simulink model "ctrl_student"  (R2020b)
settings: Solver=FixedStepAuto  StartTime=0.0  StopTime=Inf  FixedStep=0.01  RelTol=1e-3  EnableMultiTasking=on
model workspace (MAT data in the model file):
  SL_ROS_VariableLengthArrays_MaxSizes.CommonInfo.ArrayTruncateAction = 'EmitWarning'
  SL_ROS_VariableLengthArrays_MaxSizes.MsgTypeMap = containers.Map
  SL_ROS_VariableLengthArrays_MaxSizes.MsgTypeMap.serialization.keys = {'std_msgs/MultiArrayDimension', 'std_msgs/MultiArrayLayout'}
  SL_ROS_VariableLengthArrays_MaxSizes.MsgTypeMap.serialization.values{1}.PropertyName = 'Label'
  SL_ROS_VariableLengthArrays_MaxSizes.MsgTypeMap.serialization.values{1}.DataType = 'uint8'
  SL_ROS_VariableLengthArrays_MaxSizes.MsgTypeMap.serialization.values{1}.MaxLength = 2
  SL_ROS_VariableLengthArrays_MaxSizes.MsgTypeMap.serialization.values{2}.PropertyName = 'Dim'
  SL_ROS_VariableLengthArrays_MaxSizes.MsgTypeMap.serialization.values{2}.DataType = 'std_msgs/MultiArrayDimension'
  SL_ROS_VariableLengthArrays_MaxSizes.MsgTypeMap.serialization.values{2}.MaxLength = 1
  SL_ROS_VariableLengthArrays_MaxSizes.MsgTypeMap.serialization.uniformity = 0
  SL_ROS_VariableLengthArrays_MaxSizes.MsgTypeMap.serialization.keyType = 'char'
  SL_ROS_VariableLengthArrays_MaxSizes.MsgTypeMap.serialization.valueType = 'any'
undefined symbols (not defined in the file): Data, Data_SL_Info, Layout, X, Y, Z
libraries: robotlib x12
settings Model: SimulationMode=external  ExtModeEnableFloating=off  Creator=erlendbasso  LastModifiedBy=erlendbasso
settings SolverCC: PositivePriorityOrder=on
settings OptimizationCC: EnhancedBackFolding=on  PassReuseOutputArgsAs=Individual arguments  ZeroExternalMemoryAtStartup=off  ZeroInternalMemoryAtStartup=off  MaxStackSize=64  OptimizeBlockOrder=speed  DifferentSizesBufferReuse=on  OptimizationCustomize=off  EfficientTunableParamExpr=on
settings DebuggingCC: ParameterTunabilityLossMsg=error
settings HardwareCC: ProdBitPerPointer=32  ProdBitPerSizeT=32  ProdBitPerPtrDiffT=32  ProdLargestAtomicInteger=Long  ProdLargestAtomicFloat=Double  ProdWordSize=32  ProdHWDeviceType=ARM Compatible->ARM Cortex
settings RTWCC: Description=Embedded Coder  SystemTargetFile=ert.tlc  HardwareBoard=Raspberry Pi - Robot Operating System (ROS)  TLCOptions="-aInlineSetEventsForThisBaseRateFcn=TLC_FALSE -aSuppressMultiTaskScheduler=TLC_FALSE  -aRateBasedStepFcn=0"  TemplateMakefile=ert_default_tmf  Toolchain=Catkin  BuildConfiguration=Faster Runs  TargetLang=C++
settings CodeAppCC: ForceParamTrailComments=on  IgnoreCustomStorageClasses=off  OperatorAnnotations=on  SimulinkDataObjDesc=on  SFDataObjDesc=on  InsertBlockDesc=on
settings ERTTargetCC: SupportContinuousTime=on  SupportVariableSizeSignals=on  ExtModeTransport=2  ExtModeMexFile=ext_xcp  ExtModeIntrfLevel=Level2 - Open

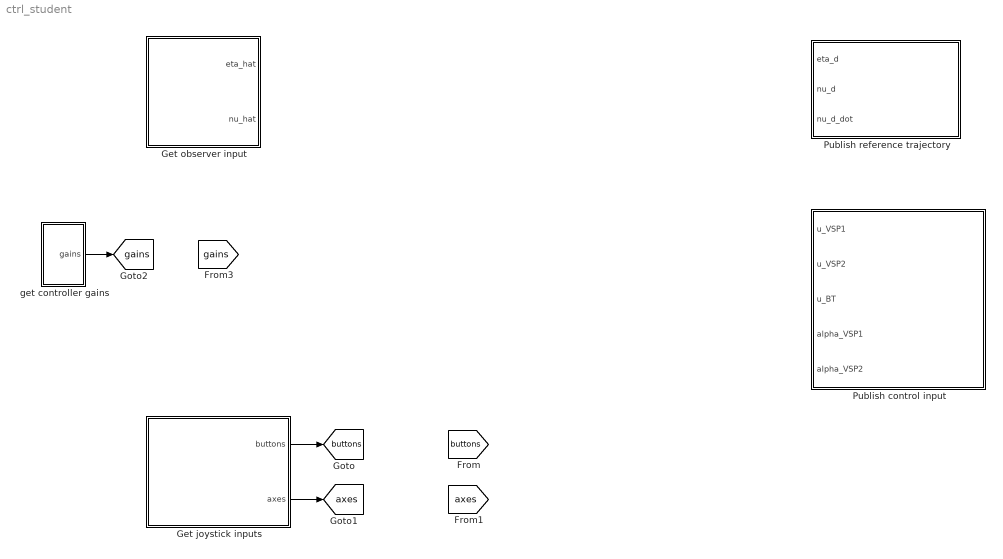
== system ctrl_student ==
  Get joystick inputs : Subsystem
  Get observer input : Subsystem
  Publish control input : Subsystem
  Publish reference trajectory : Subsystem
  get controller gains : Subsystem
  tag scope: axes=global, buttons=global, gains=global
  wires:
  Get joystick inputs/2(axes) -> [axes]
  Get joystick inputs/1(buttons) -> [buttons]
  get controller gains/1(gains) -> [gains]

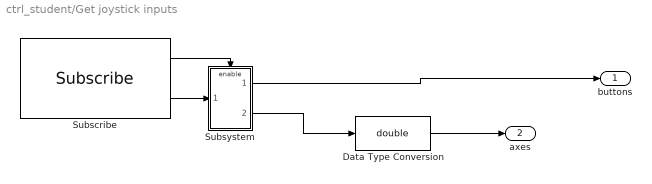
== system ctrl_student/Get joystick inputs ==
  Data Type Conversion : DataTypeConversion  OutDataTypeStr=double
  Subscribe : robotlib/Subscribe  topicSource=Select from ROS network  topic=/joy  messageType=sensor_msgs/Joy  SampleTime=0.01  legacyBusStruct=off  messageQueueLength=1
  Subsystem : Subsystem
  buttons : Outport
  axes : Outport  Port=2
  wires:
  Subscribe/1 -> Subsystem/Enable
  Subscribe/2 -> Subsystem/1(In1)
  Subsystem/2(<Axes>) -> Data Type Conversion/1
  Subsystem/1(<Buttons>) -> buttons/1
  Data Type Conversion/1 -> axes/1

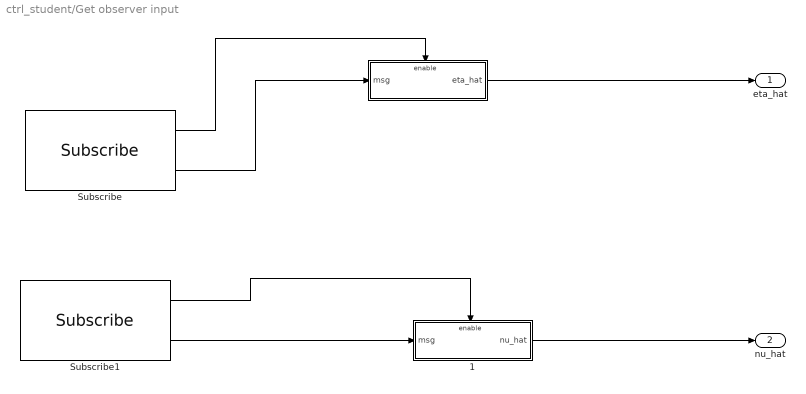
== system ctrl_student/Get observer input ==
  " " : Subsystem
  " 1" : Subsystem
  Subscribe : robotlib/Subscribe  topicSource=Specify your own  topic=/CSEI/observer/eta  messageType=geometry_msgs/Vector3  SampleTime=0.01  legacyBusStruct=off  messageQueueLength=1
  Subscribe1 : robotlib/Subscribe  topicSource=Specify your own  topic=/CSEI/observer/nu  messageType=geometry_msgs/Vector3  SampleTime=0.01  legacyBusStruct=off  messageQueueLength=1
  eta_hat : Outport
  nu_hat : Outport  Port=2
  wires:
  " 1"/1(nu_hat) -> nu_hat/1
  " "/1(eta_hat) -> eta_hat/1
  Subscribe/1 -> " "/Enable
  Subscribe/2 -> " "/1(msg)
  Subscribe1/1 -> " 1"/Enable
  Subscribe1/2 -> " 1"/1(msg)

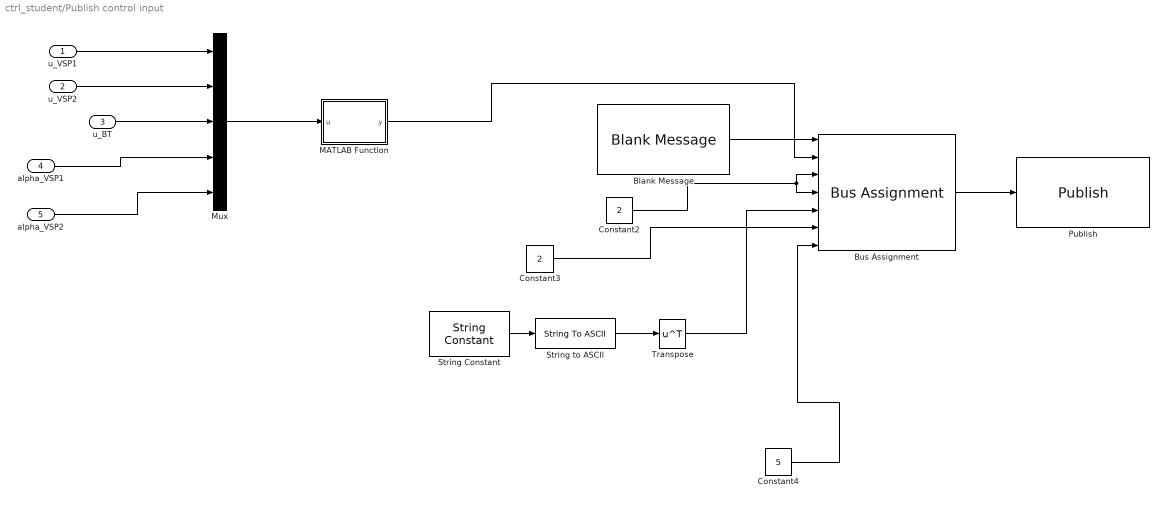
== system ctrl_student/Publish control input ==
  u_VSP1 : Inport
  u_VSP2 : Inport  Port=2
  u_BT : Inport  Port=3
  alpha_VSP1 : Inport  Port=4
  alpha_VSP2 : Inport  Port=5
  Blank Message : robotlib/Blank Message  messageClass=Message  entityType=std_msgs/Float64MultiArray  messageType=std_msgs/Float64MultiArray  SampleTime=0.01  legacyBusStruct=off
  Bus Assignment : BusAssignment  AssignedSignals=Data,Layout.Dim.Stride,Layout.Dim.Size,Layout.Dim.Label,Layout.Dim.Label_SL_Info.CurrentLength,Data_SL_Info.CurrentLength
  Constant2 : Constant  Value=2  OutDataTypeStr=uint32  SampleTime=Inf
  Constant3 : Constant  Value=2  OutDataTypeStr=uint32  SampleTime=Inf
  Constant4 : Constant  Value=5  OutDataTypeStr=uint32  SampleTime=Inf
  MATLAB Function : MATLAB Function  TreatAsAtomicUnit=on
  Mux : Mux  Inputs=5
  Publish : robotlib/Publish  topicSource=Specify your own  topic=/CSEI/u  messageType=std_msgs/Float64MultiArray  legacyBusStruct=off  messageQueueLength=1
  String Constant : StringConstant  String="\"\""
  String to ASCII : StringToASCII  OutputVectorSize=2
  Transpose : Math  Operator=transpose  SaturateOnIntegerOverflow=on
  wires:
  String Constant/1 -> String to ASCII/1
  Transpose/1 -> Bus Assignment/5
  Bus Assignment/1 -> Publish/1
  Constant3/1 -> Bus Assignment/6
  Constant2/1 -> Bus Assignment/3, Bus Assignment/4
  String to ASCII/1 -> Transpose/1
  Constant4/1 -> Bus Assignment/7
  Blank Message/1 -> Bus Assignment/1
  MATLAB Function/1(y) -> Bus Assignment/2
  alpha_VSP2/1 -> Mux/5
  Mux/1 -> MATLAB Function/1(u)
  alpha_VSP1/1 -> Mux/4
  u_BT/1 -> Mux/3
  u_VSP1/1 -> Mux/1
  u_VSP2/1 -> Mux/2

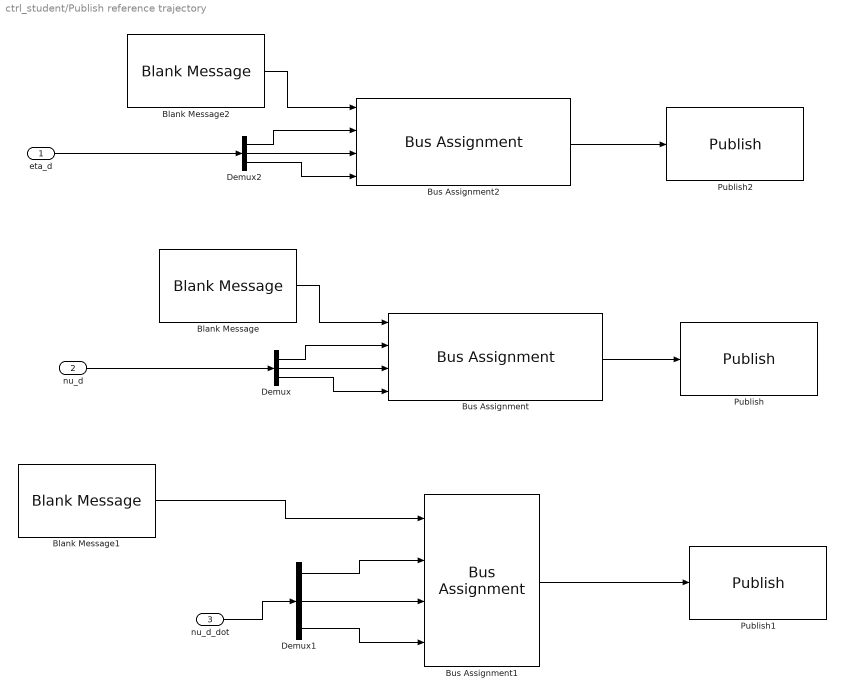
== system ctrl_student/Publish reference trajectory ==
  eta_d : Inport
  nu_d : Inport  Port=2
  nu_d_dot : Inport  Port=3
  Blank Message : robotlib/Blank Message  messageClass=Message  entityType=geometry_msgs/Vector3  messageType=geometry_msgs/Vector3  SampleTime=0.01  legacyBusStruct=off
  Blank Message1 : robotlib/Blank Message  messageClass=Message  entityType=geometry_msgs/Vector3  messageType=geometry_msgs/Vector3  SampleTime=0.01  legacyBusStruct=off
  Blank Message2 : robotlib/Blank Message  messageClass=Message  entityType=geometry_msgs/Vector3  messageType=geometry_msgs/Vector3  SampleTime=0.01  legacyBusStruct=off
  Bus Assignment : BusAssignment  AssignedSignals=X,Y,Z
  Bus Assignment1 : BusAssignment  AssignedSignals=X,Y,Z
  Bus Assignment2 : BusAssignment  AssignedSignals=X,Y,Z
  Demux : Demux  Outputs=3
  Demux1 : Demux  Outputs=3
  Demux2 : Demux  Outputs=3
  Publish : robotlib/Publish  topicSource=Specify your own  topic=/CSEI/ref/nu_d  messageType=geometry_msgs/Vector3  legacyBusStruct=off  messageQueueLength=1
  Publish1 : robotlib/Publish  topicSource=Specify your own  topic=/CSEI/ref/nu_d_dot  messageType=geometry_msgs/Vector3  legacyBusStruct=off  messageQueueLength=1
  Publish2 : robotlib/Publish  topicSource=Specify your own  topic=/CSEI/ref/eta_d  messageType=geometry_msgs/Vector3  legacyBusStruct=off  messageQueueLength=1
  wires:
  Demux/1 -> Bus Assignment/2
  Bus Assignment/1 -> Publish/1
  nu_d/1 -> Demux/1
  Demux/2 -> Bus Assignment/3
  Blank Message/1 -> Bus Assignment/1
  Demux/3 -> Bus Assignment/4
  Demux1/2 -> Bus Assignment1/3
  Bus Assignment1/1 -> Publish1/1
  Blank Message1/1 -> Bus Assignment1/1
  Demux1/1 -> Bus Assignment1/2
  Demux1/3 -> Bus Assignment1/4
  nu_d_dot/1 -> Demux1/1
  eta_d/1 -> Demux2/1
  Bus Assignment2/1 -> Publish2/1
  Blank Message2/1 -> Bus Assignment2/1
  Demux2/3 -> Bus Assignment2/4
  Demux2/1 -> Bus Assignment2/2
  Demux2/2 -> Bus Assignment2/3

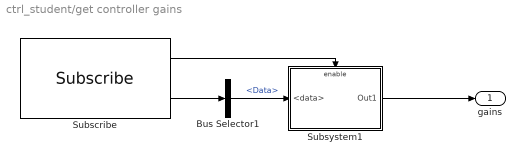
== system ctrl_student/get controller gains ==
  Bus Selector1 : BusSelector  OutputSignals=Data
  Subscribe : robotlib/Subscribe  topicSource=Specify your own  topic=/CSEI/controller/gains  messageType=std_msgs/Float64MultiArray  SampleTime=0.01  legacyBusStruct=off  messageQueueLength=1
  Subsystem1 : Subsystem
  gains : Outport
  wires:
  Subsystem1/1(Out1) -> gains/1
  Subscribe/1 -> Subsystem1/Enable
  Subscribe/2 -> Bus Selector1/1
  Bus Selector1/1 -> Subsystem1/1(<data>)  "<Data>"

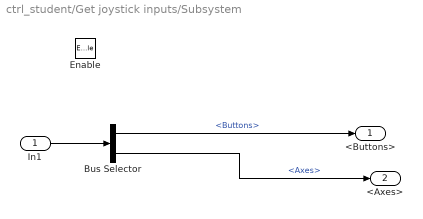
== system ctrl_student/Get joystick inputs/Subsystem ==
  In1 : Inport
  Enable : EnablePort
  Bus Selector : BusSelector  OutputSignals=Buttons,Axes
  <Buttons> : Outport
  <Axes> : Outport  Port=2
  wires:
  In1/1 -> Bus Selector/1
  Bus Selector/1 -> <Buttons>/1  "<Buttons>"
  Bus Selector/2 -> <Axes>/1  "<Axes>"

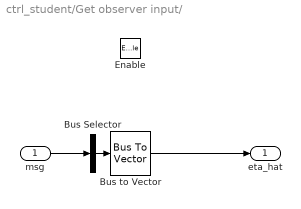
== system ctrl_student/Get observer input/  ==
  msg : Inport
  Enable : EnablePort
  Bus Selector : BusSelector  OutputSignals=X,Y,Z  OutputAsBus=on
  Bus to Vector : BusToVector
  eta_hat : Outport
  wires:
  msg/1 -> Bus Selector/1
  Bus to Vector/1 -> eta_hat/1
  Bus Selector/1 -> Bus to Vector/1

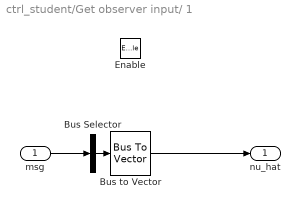
== system ctrl_student/Get observer input/ 1 ==
  msg : Inport
  Enable : EnablePort
  Bus Selector : BusSelector  OutputSignals=X,Y,Z  OutputAsBus=on
  Bus to Vector : BusToVector
  nu_hat : Outport
  wires:
  msg/1 -> Bus Selector/1
  Bus to Vector/1 -> nu_hat/1
  Bus Selector/1 -> Bus to Vector/1

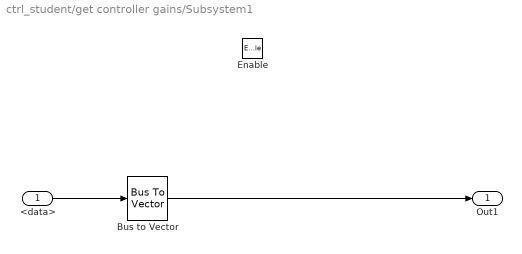
== system ctrl_student/get controller gains/Subsystem1 ==
  <data> : Inport
  Enable : EnablePort
  Bus to Vector : BusToVector
  Out1 : Outport
  wires:
  Bus to Vector/1 -> Out1/1
  <data>/1 -> Bus to Vector/1

== matlab function ctrl_student/Publish control input/MATLAB Function ==
  data: u input; y output
function y = fcn(u)
y = zeros(128,1);

y(1:size(u,1)) = u;
